simulink model "pitch_control"  (R2021b)
settings: Solver=VariableStepAuto  StartTime=0.0  StopTime=40  RelTol=1e-3
settings Model: Creator=Abner Souza  LastModifiedBy=Abner Souza

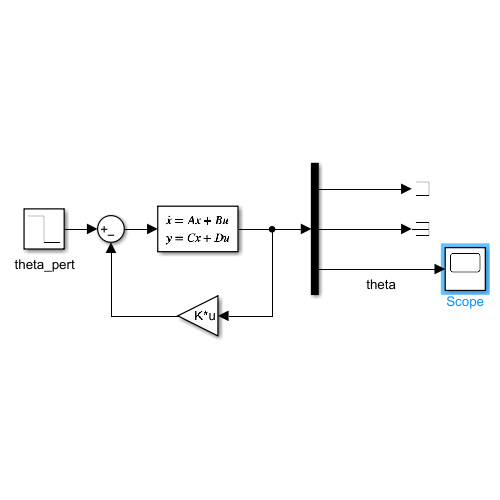
[thumbnail: Simulink's stored preview of the top-level diagram]
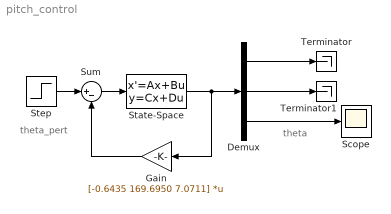
== system pitch_control ==
  note: theta_pert
  note: theta
  Demux : Demux  Outputs=3
  Gain : Gain  Gain=[-0.6435 169.6950 7.0711]  Multiplication=Matrix(K*u)
  Scope : Scope
  State-Space : StateSpace  A=[-0.313 56.7 0; -0.0139 -0.426 0; 0 56.7 0]  B=[0.232; 0.0203; 0]  C=eye(3)  D=[0;0;0]  InitialCondition=0  ContinuousStateAttributes={'Angle_of_attack', 'Pitch_rate', 'Pitch_angle'}
  Step : Step  Time=0  After=-0.25  SampleTime=0
  Sum : Sum  Inputs=|+-
  Terminator : Terminator
  Terminator1 : Terminator
  wires:
  State-Space/1 -> Gain/1, Demux/1
  Demux/2 -> Terminator1/1
  Demux/1 -> Terminator/1
  Demux/3 -> Scope/1
  Step/1 -> Sum/1
  Sum/1 -> State-Space/1
  Gain/1 -> Sum/2
